simulink model "otch_5_0"  (R2017b)
settings: Solver=VariableStepAuto  StartTime=0.0  StopTime=4.5  RelTol=1e-3
settings Model: Creator=anton  LastModifiedBy=anton

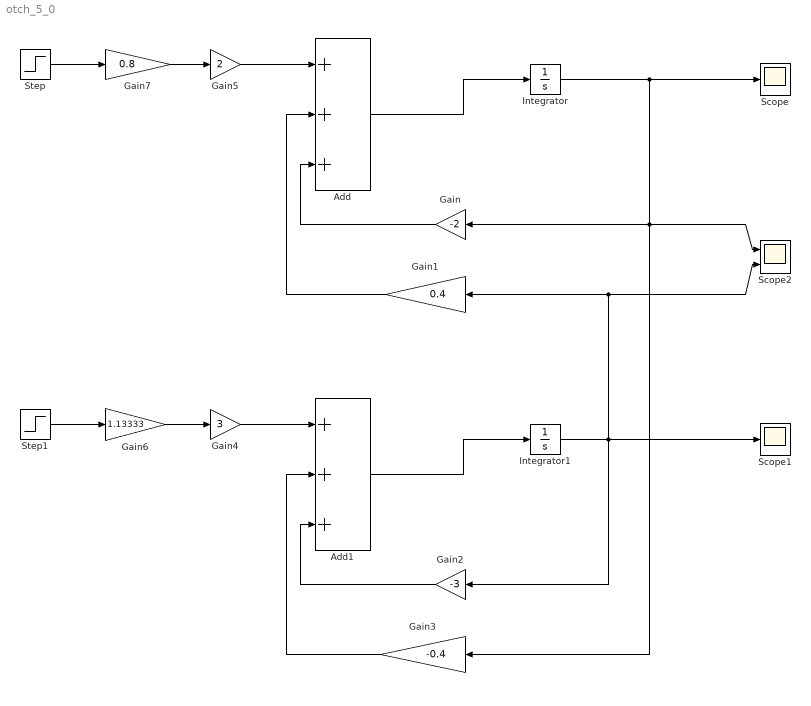
== system otch_5_0 ==
  Add : Sum  Inputs=+++
  Add1 : Sum  Inputs=+++
  Gain : Gain  Gain=-2
  Gain1 : Gain  Gain=0.4
  Gain2 : Gain  Gain=-3
  Gain3 : Gain  Gain=-0.4
  Gain4 : Gain  Gain=3
  Gain5 : Gain  Gain=2
  Gain6 : Gain  Gain=1.13333
  Gain7 : Gain  Gain=0.8
  Integrator : Integrator
  Integrator1 : Integrator
  Scope : Scope
  Scope1 : Scope
  Scope2 : Scope  NumInputPorts=2
  Step : Step  Time=0  After=1.7  SampleTime=0
  Step1 : Step  Time=0  After=1.7  SampleTime=0
  wires:
  Add/1 -> Integrator/1
  Gain/1 -> Add/3
  Gain1/1 -> Add/2
  Gain2/1 -> Add1/3
  Gain3/1 -> Add1/2
  Integrator1/1 -> Scope1/1, Gain2/1, Scope2/2, Gain1/1
  Add1/1 -> Integrator1/1
  Step1/1 -> Gain6/1
  Gain4/1 -> Add1/1
  Gain5/1 -> Add/1
  Step/1 -> Gain7/1
  Integrator/1 -> Scope2/1, Gain3/1, Gain/1, Scope/1
  Gain6/1 -> Gain4/1
  Gain7/1 -> Gain5/1
